simulink model "block_diagram"  (R2025a)
settings: Solver=VariableStepAuto  StartTime=0.0  StopTime=2  FixedStep=1e-4  RelTol=1e-2  AbsTol=1e-5
values from neighbouring files (symbols this model uses):
  Kjt = 1/n2 * 1/n1    [main.m]
  Ktj = 1/Kjt    [main.m]
  nKm = Km    [main.m]
  yd = 0.04    [main.m]
  Ye = 1/(s*Lw + Rw)    [main.m]
  Ym = Ztot    [main.m]
settings Model: Creator=flipa  LastModifiedBy=flipa

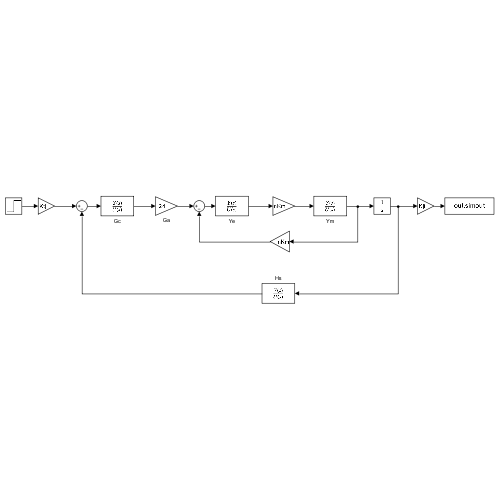
[thumbnail: Simulink's stored preview of the top-level diagram]
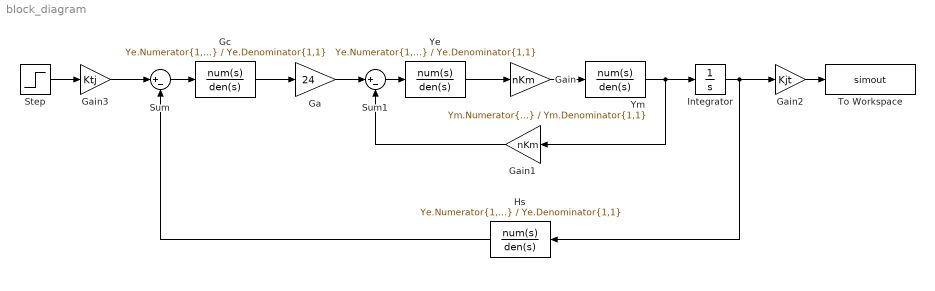
== system block_diagram ==
  Ga : Gain  Gain=24
  Gain : Gain  Gain=nKm
  Gain1 : Gain  Gain=nKm
  Gain2 : Gain  Gain=Kjt
  Gain3 : Gain  Gain=Ktj
  Gc : TransferFcn  Numerator=Ye.Numerator{1,1}  Denominator=Ye.Denominator{1,1}  ContinuousStateAttributes='iw'
  Hs : TransferFcn  Numerator=Ye.Numerator{1,1}  Denominator=Ye.Denominator{1,1}  ContinuousStateAttributes='iw'
  Integrator : Integrator
  Step : Step  Time=0  After=yd  SampleTime=0
  Sum : Sum  Inputs=|+-
  Sum1 : Sum  Inputs=|+-
  To Workspace : ToWorkspace  VariableName=simout  SaveFormat=Timeseries  SampleTime=-1
  Ye : TransferFcn  Numerator=Ye.Numerator{1,1}  Denominator=Ye.Denominator{1,1}  ContinuousStateAttributes='iw'
  Ym : TransferFcn  Numerator=Ym.Numerator{1,1}  Denominator=Ym.Denominator{1,1}  ContinuousStateAttributes='iw'
  wires:
  Gain1/1 -> Sum1/2
  Sum1/1 -> Ye/1
  Gain2/1 -> To Workspace/1
  Step/1 -> Gain3/1
  Gain3/1 -> Sum/1
  Ga/1 -> Sum1/1
  Sum/1 -> Gc/1
  Gc/1 -> Ga/1
  Ye/1 -> Gain/1
  Integrator/1 -> Hs/1, Gain2/1
  Hs/1 -> Sum/2
  Gain/1 -> Ym/1
  Ym/1 -> Gain1/1, Integrator/1
